simulink model "phase_test"  (R2015b)
settings: Solver=VariableStepAuto  StartTime=0.0  StopTime=0.25  RelTol=1e-3
settings Model: Creator=YogurtSuee  LastModifiedBy=YogurtSuee

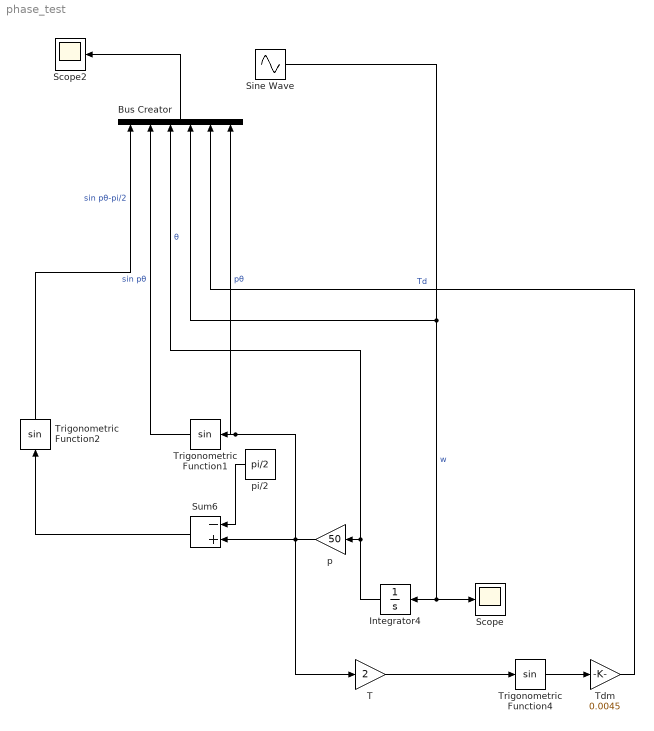
== system phase_test ==
  Bus Creator : BusCreator  Inputs=6
  Integrator4 : Integrator
  Scope : Scope
  Scope2 : Scope
  Sine Wave : Sin  Frequency=50  SampleTime=0
  Sum6 : Sum  Inputs=-+
  T : Gain  Gain=2
  Tdm : Gain  Gain=0.0045
  Trigonometric Function1 : Trigonometry
  Trigonometric Function2 : Trigonometry
  Trigonometric Function4 : Trigonometry
  p : Gain  Gain=50
  pi/2 : Constant  Value=pi/2
  wires:
  Tdm/1 -> Bus Creator/5  "Td"
  Sine Wave/1 -> Bus Creator/4, Integrator4/1, Scope/1  "w"
  Integrator4/1 -> p/1, Bus Creator/3  "θ"
  p/1 -> Bus Creator/6, Trigonometric Function1/1, Sum6/2, T/1  "pθ"
  pi/2/1 -> Sum6/1
  Trigonometric Function4/1 -> Tdm/1
  T/1 -> Trigonometric Function4/1
  Bus Creator/1 -> Scope2/1
  Trigonometric Function1/1 -> Bus Creator/2  "sin pθ"
  Sum6/1 -> Trigonometric Function2/1
  Trigonometric Function2/1 -> Bus Creator/1  "sin pθ-pi/2"
